simulink model "SetPointWeighting"  (Simulink 10.3)
settings: Solver=ode4  StartTime=0.0  StopTime=40  FixedStep=0.01  RelTol=1e-3
undefined symbols (not defined in the file or in its folder): sigbuilder_block
settings Model: Creator=Mertcan  LastModifiedBy=Mertcan
settings SolverCC: AlgebraicLoopSolver=Auto
settings DataIOCC: SaveFormat=Dataset  SignalLoggingSaveFormat=Dataset  ReturnWorkspaceOutputs=on
settings OptimizationCC: ExpressionDepthLimit=128  LifeSpan=auto
settings DebuggingCC: UnderspecifiedInitializationDetection=Simplified  MergeDetectMultiDrivingBlocksExec=error  FcnCallInpInsideContextMsg=error  StateNameClashWarn=none  SFUnexpectedBacktrackingDiag=error  SFNoUnconditionalDefaultTransitionDiag=error  SFExecutionAtInitializationDiag=warning  SFMachineParentedDataDiag=error  ArithmeticOperatorsInVariantConditions=error
settings HardwareCC: ProdBitPerPointer=64  ProdBitPerSizeT=64  ProdBitPerPtrDiffT=64  ProdLargestAtomicFloat=Float  ProdIntDivRoundTo=Zero  ProdEndianess=LittleEndian  ProdWordSize=64  ProdHWDeviceType=Intel->x86-64 (Windows64)
settings ModelReferenceCC: PropagateSignalLabelsOutOfModel=on
settings SFSimCC: SimUseLocalCustomCode=on  CustomCodeUndefinedFunction=FilterOut
settings RTWCC: RTWUseLocalCustomCode=on
settings CodeAppCC: StateflowObjectComments=off
settings GRTTargetCC: TargetLangStandard=C99 (ISO)  CombineOutputUpdateFcns=on  GRTInterface=off
settings ConfigComp: CovMetricSettings=dwe  CovSaveCumulativeToWorkspaceVar=off  CovSaveSingleToWorkspaceVar=off  CovExternalEMLEnable=on

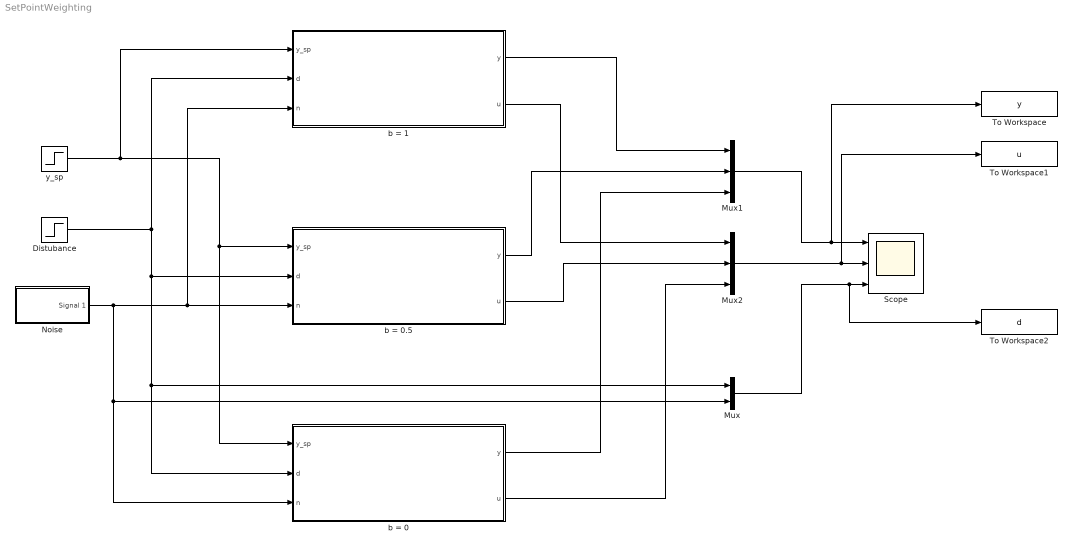
== system SetPointWeighting ==
  Distubance : Step  Time=15  After=-1  SampleTime=0
  Mux : Mux  Inputs=2
  Mux1 : Mux  Inputs=3
  Mux2 : Mux  Inputs=3
  Noise : Subsystem  Tag=STV Subsys  LoadFcn=sigbuilder_block('load');  StartFcn=sigbuilder_block('start');  StopFcn=sigbuilder_block('stop');  ClipboardFcn=sigbuilder_block('clipboard');  mask(Sigbuilder block){tuvar=[0:10]}
      mask help: Simulink:masks:SigbuilderBlock_MD
      mask init:
      | if ~strcmp(get_param(bdroot(gcbh),'SimulationStatus'),'stopped') tuvar = sigbuilder_block('maskInit'); end
      settings: CopyFcn=sigbuilder_block('copy');  DeleteFcn=sigbuilder_block('delete');  ModelCloseFcn=sigbuilder_block('modelClose');  PreSaveFcn=sigbuilder_block('preSave');  PauseFcn=sigbuilder_block('pause');  ContinueFcn=sigbuilder_block('continue');  NameChangeFcn=sigbuilder_block('namechange');  OpenFcn=sigbuilder_block('open',[-243.75 876 960 452.25 ]);  CloseFcn=sigbuilder_block('close');
      mask Display: plot(0, 0, 100, 100,[2, 2, 32, 32, 2], [68, 8, 8, 68, 68],[32, 2], [38, 38], [32, 19, 2],[53, 60, 44], [32, 17, 17, 2],[16, 16, 31, 31]);txt = getActiveGroup(gcbh);text(2, 100, txt,'verticalAlignment', 'top');
  Scope : Scope  NumInputPorts=3
  To Workspace : ToWorkspace  VariableName=y  SaveFormat=Timeseries  SampleTime=-1
  To Workspace1 : ToWorkspace  VariableName=u  SaveFormat=Timeseries  SampleTime=-1
  To Workspace2 : ToWorkspace  VariableName=d  SaveFormat=Timeseries  SampleTime=-1
  b = 0 : Subsystem
  b = 0.5 : Subsystem
  b = 1 : Subsystem
  y_sp : Step  Time=0  Before=1  SampleTime=0
  wires:
  y_sp/1 -> b = 0/1(y_sp), b = 0.5/1(y_sp), b = 1/1(y_sp)
  Distubance/1 -> b = 1/2(d), Mux/1, b = 0/2(d), b = 0.5/2(d)
  Noise/1(Signal 1) -> Mux/2, b = 0/3(n), b = 0.5/3(n), b = 1/3(n)
  Mux1/1 -> To Workspace/1, Scope/1
  Mux2/1 -> To Workspace1/1, Scope/2
  Mux/1 -> To Workspace2/1, Scope/3
  b = 1/1(y) -> Mux1/1
  b = 1/2(u) -> Mux2/1
  b = 0.5/1(y) -> Mux1/2
  b = 0.5/2(u) -> Mux2/2
  b = 0/1(y) -> Mux1/3
  b = 0/2(u) -> Mux2/3

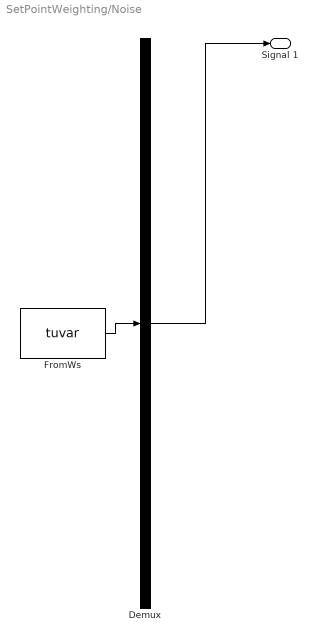
== system SetPointWeighting/Noise ==
  Demux : Demux  Tag=STV Demux  Outputs=1
      settings: DisplayOption=none
  FromWs : FromWorkspace  Tag=STV FromWs  VariableName=tuvar  SigBuilderData=DataTag0  VnvData=DataTag1
      SigBuilderData=|
      | common.afterFinalStr = 'Extrapolate'
      | common.sampleTime = 0
      | dataSet.timeRange = [0 40]
      | dataSet.name = 'Group 1'
      | sbobj.Groups.Name = 'Group 1'
      | sbobj.Groups.Signals.Name = 'Signal 1'
      | sbobj.Groups.Signals.XData = [0 29 30 31 40]
      | sbobj.Groups.Signals.YData = [0 0 0.1 0 0]
      | sbobj.Groups.TimeRange = [0 40]
  Signal 1 : Outport  Tag=STV Outport
  wires:
  Demux/1 -> Signal 1/1
  FromWs/1 -> Demux/1

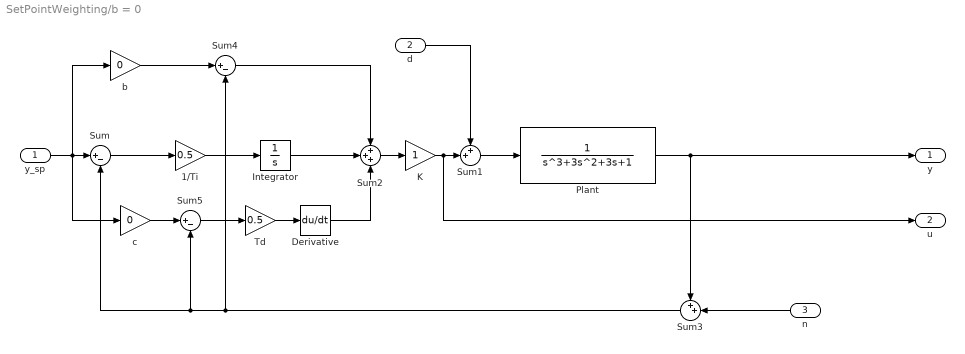
== system SetPointWeighting/b = 0 ==
  y_sp : Inport
  d : Inport  Port=2
  n : Inport  Port=3
  1/Ti : Gain  Gain=0.5
  Derivative : Derivative
  Integrator : Integrator
  K : Gain
  Plant : TransferFcn  Denominator=[1 3 3 1]
  Sum : Sum  Inputs=|+-
  Sum1 : Sum  Inputs=++|
  Sum2 : Sum  Inputs=+++
  Sum3 : Sum  Inputs=++|
  Sum4 : Sum  Inputs=|+-
  Sum5 : Sum  Inputs=|+-
  Td : Gain  Gain=0.5
  b : Gain  Gain=0
  c : Gain  Gain=0
  y : Outport
  u : Outport  Port=2
  wires:
  K/1 -> u/1, Sum1/2
  Td/1 -> Derivative/1
  Derivative/1 -> Sum2/3
  Sum4/1 -> Sum2/1
  Sum2/1 -> K/1
  b/1 -> Sum4/1
  Sum/1 -> 1/Ti/1
  Integrator/1 -> Sum2/2
  Sum5/1 -> Td/1
  Sum1/1 -> Plant/1
  y_sp/1 -> c/1, b/1, Sum/1
  Plant/1 -> y/1, Sum3/1
  1/Ti/1 -> Integrator/1
  c/1 -> Sum5/1
  Sum3/1 -> Sum5/2, Sum/2, Sum4/2
  n/1 -> Sum3/2
  d/1 -> Sum1/1

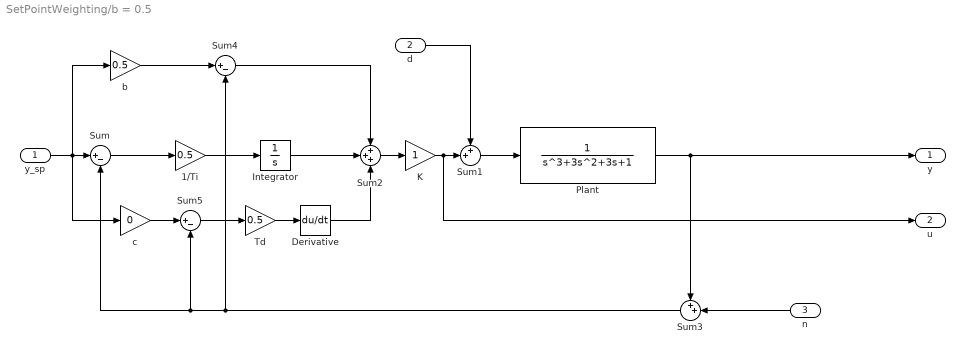
== system SetPointWeighting/b = 0.5 ==
  y_sp : Inport
  d : Inport  Port=2
  n : Inport  Port=3
  1/Ti : Gain  Gain=0.5
  Derivative : Derivative
  Integrator : Integrator
  K : Gain
  Plant : TransferFcn  Denominator=[1 3 3 1]
  Sum : Sum  Inputs=|+-
  Sum1 : Sum  Inputs=++|
  Sum2 : Sum  Inputs=+++
  Sum3 : Sum  Inputs=++|
  Sum4 : Sum  Inputs=|+-
  Sum5 : Sum  Inputs=|+-
  Td : Gain  Gain=0.5
  b : Gain  Gain=0.5
  c : Gain  Gain=0
  y : Outport
  u : Outport  Port=2
  wires:
  d/1 -> Sum1/1
  n/1 -> Sum3/2
  Sum3/1 -> Sum4/2, Sum/2, Sum5/2
  c/1 -> Sum5/1
  1/Ti/1 -> Integrator/1
  Plant/1 -> Sum3/1, y/1
  y_sp/1 -> Sum/1, b/1, c/1
  Sum1/1 -> Plant/1
  Sum5/1 -> Td/1
  Integrator/1 -> Sum2/2
  Sum/1 -> 1/Ti/1
  b/1 -> Sum4/1
  Sum2/1 -> K/1
  Sum4/1 -> Sum2/1
  Derivative/1 -> Sum2/3
  Td/1 -> Derivative/1
  K/1 -> Sum1/2, u/1

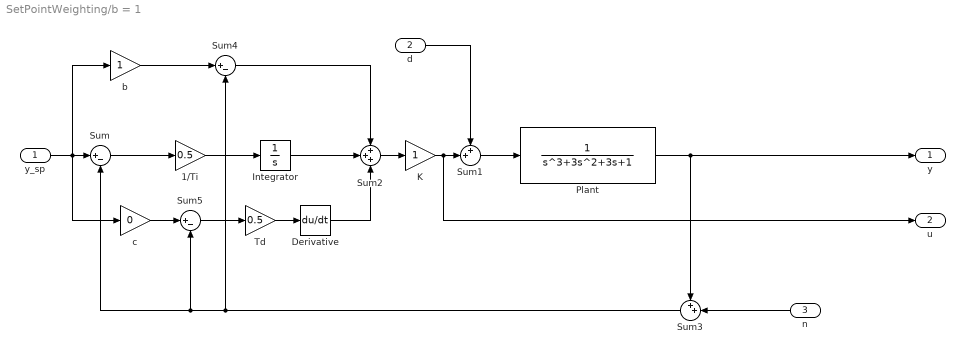
== system SetPointWeighting/b = 1 ==
  y_sp : Inport
  d : Inport  Port=2
  n : Inport  Port=3
  1/Ti : Gain  Gain=0.5
  Derivative : Derivative
  Integrator : Integrator
  K : Gain
  Plant : TransferFcn  Denominator=[1 3 3 1]
  Sum : Sum  Inputs=|+-
  Sum1 : Sum  Inputs=++|
  Sum2 : Sum  Inputs=+++
  Sum3 : Sum  Inputs=++|
  Sum4 : Sum  Inputs=|+-
  Sum5 : Sum  Inputs=|+-
  Td : Gain  Gain=0.5
  b : Gain
  c : Gain  Gain=0
  y : Outport
  u : Outport  Port=2
  wires:
  K/1 -> u/1, Sum1/2
  Td/1 -> Derivative/1
  Derivative/1 -> Sum2/3
  Sum4/1 -> Sum2/1
  Sum2/1 -> K/1
  b/1 -> Sum4/1
  Sum/1 -> 1/Ti/1
  Integrator/1 -> Sum2/2
  Sum5/1 -> Td/1
  Sum1/1 -> Plant/1
  y_sp/1 -> c/1, b/1, Sum/1
  Plant/1 -> y/1, Sum3/1
  1/Ti/1 -> Integrator/1
  c/1 -> Sum5/1
  Sum3/1 -> Sum5/2, Sum/2, Sum4/2
  n/1 -> Sum3/2
  d/1 -> Sum1/1
